simulink model "Tut13_AtomicSubsystem_Part1"  (R2021a)
settings: Solver=FixedStepDiscrete  StartTime=0.0  StopTime=20  FixedStep=1  MaxStep=1  RelTol=1e-3
settings Model: Creator=cheta  LastModifiedBy=cheta

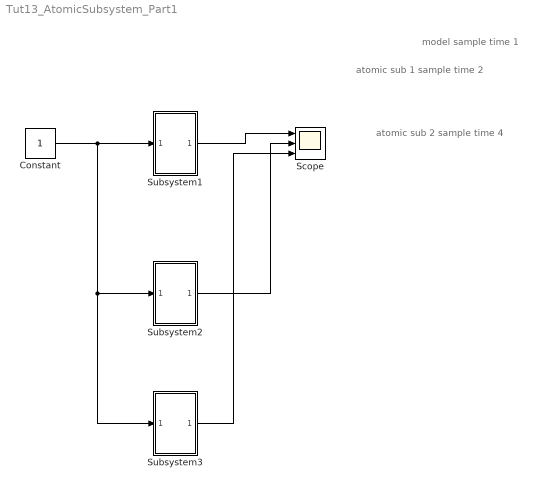
== system Tut13_AtomicSubsystem_Part1 ==
  note: atomic sub 2 sample time 4
  note: atomic sub 1 sample time 2
  note: model sample time 1
  Constant : Constant
  Scope : Scope  NumInputPorts=3
  Subsystem1 : Subsystem
  Subsystem2 : Subsystem  TreatAsAtomicUnit=on  SystemSampleTime=0.5
  Subsystem3 : Subsystem  TreatAsAtomicUnit=on  SystemSampleTime=4
  wires:
  Constant/1 -> Subsystem3/1(In1), Subsystem2/1(In1), Subsystem1/1(In1)
  Subsystem1/1(Out1) -> Scope/1
  Subsystem2/1(Out1) -> Scope/2
  Subsystem3/1(Out1) -> Scope/3

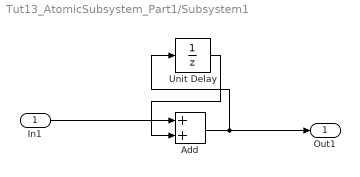
== system Tut13_AtomicSubsystem_Part1/Subsystem1 ==
  In1 : Inport
  Add : Sum
  Unit Delay : UnitDelay  SampleTime=-1  HasFrameUpgradeWarning=on
  Out1 : Outport
  wires:
  Unit Delay/1 -> Add/2
  Add/1 -> Out1/1, Unit Delay/1
  In1/1 -> Add/1

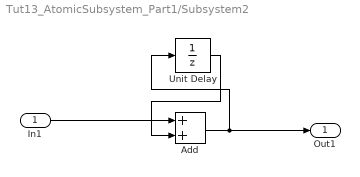
== system Tut13_AtomicSubsystem_Part1/Subsystem2 ==
  In1 : Inport
  Add : Sum
  Unit Delay : UnitDelay  SampleTime=-1  HasFrameUpgradeWarning=on
  Out1 : Outport
  wires:
  In1/1 -> Add/1
  Add/1 -> Unit Delay/1, Out1/1
  Unit Delay/1 -> Add/2

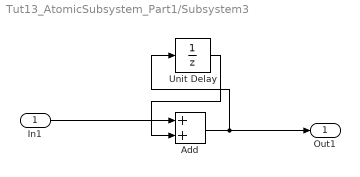
== system Tut13_AtomicSubsystem_Part1/Subsystem3 ==
  In1 : Inport
  Add : Sum
  Unit Delay : UnitDelay  SampleTime=-1  HasFrameUpgradeWarning=on
  Out1 : Outport
  wires:
  Unit Delay/1 -> Add/2
  Add/1 -> Out1/1, Unit Delay/1
  In1/1 -> Add/1
